simulink library "Lib_EMTAT"  (R2023b)
settings: Solver=VariableStepAuto  StartTime=0.0  StopTime=10.0  RelTol=1e-3
undefined symbols (not defined in the file): MWS
libraries: simulink x34
(part 3 of 4)

== system Lib_EMTAT/Components/Power Flow/AC-DC Rectifier (Efficiency Map)/Open Circuit// Degradation Failure ==
  Eff : Inport
  DegFail? : Inport  Port=2
  OCFail? : Inport  Port=3
  Deg : Inport  Port=4
  Constant : Constant  Value=eps
  Constant1 : Constant
  Divide : Product  Inputs=**
  "If degradation failure, scale Eff." : Switch  Criteria=u2 > Threshold  SaturateOnIntegerOverflow=off  InputSameDT=off
  "If open circuit failure, set Eff = eps." : Switch  Criteria=u2 > Threshold  SaturateOnIntegerOverflow=off  InputSameDT=off
  Sum : Sum  Inputs=+-|
  "Eff " : Outport
  wires:
  DegFail?/1 -> "If degradation failure, scale Eff."/2
  "If degradation failure, scale Eff."/1 -> "If open circuit failure, set Eff = eps."/3
  Divide/1 -> "If degradation failure, scale Eff."/1
  "If open circuit failure, set Eff = eps."/1 -> "Eff "/1
  OCFail?/1 -> "If open circuit failure, set Eff = eps."/2
  Constant/1 -> "If open circuit failure, set Eff = eps."/1
  Sum/1 -> Divide/1
  Eff/1 -> "If degradation failure, scale Eff."/3, Divide/2
  Deg/1 -> Sum/2
  Constant1/1 -> Sum/1

== system Lib_EMTAT/Components/Power Flow/AC-DC Rectifier (Power Loss Map)/Compensate for Divide By Zero. ==
  note: If Vin is not equal to zero, use its value.
      | If Vin is equal to zero, it will calculate a nan value for Iin. Set Iin to zero.
  PEquivAC : Inport
  V_LN_rms : Inport  Port=2
  Fix Divide By Zero. : Subsystem
  I_L_rms : Outport
  wires:
  Fix Divide By Zero./1(I_L_rms) -> I_L_rms/1
  PEquivAC/1 -> Fix Divide By Zero./2(PEquivAC)
  V_LN_rms/1 -> Fix Divide By Zero./1(V_LN_rms)

== system Lib_EMTAT/Components/Power Flow/AC-DC Rectifier (Power Loss Map)/Direction Determination ==
  P_DC : Inport
  Ploss : Inport  Port=2
  Add1 : Sum  Inputs=-+
  Switch : Switch  Criteria=u2 ~= 0  SaturateOnIntegerOverflow=off  InputSameDT=off
  PEquivAC : Outport
  wires:
  P_DC/1 -> Switch/3, Switch/2, Add1/2
  Ploss/1 -> Add1/1
  Add1/1 -> Switch/1
  Switch/1 -> PEquivAC/1

== system Lib_EMTAT/Components/Power Flow/AC-DC Rectifier (Power Loss Map)/Efficiency ==
  P_AC : Inport
  P_DC : Inport  Port=2
  Abs : Abs  SaturateOnIntegerOverflow=off
  Abs1 : Abs  SaturateOnIntegerOverflow=off
  Fix Divide By Zero. : Subsystem
  Fix Divide By Zero.1 : Subsystem
  GreaterThan : RelationalOperator  OutDataTypeStr=boolean  RndMeth=Simplest  InputSameDT=off
  Switch : Switch  Criteria=u2 > Threshold  SaturateOnIntegerOverflow=off  InputSameDT=off
  Eff : Outport
  wires:
  Switch/1 -> Eff/1
  GreaterThan/1 -> Switch/2
  Abs1/1 -> Fix Divide By Zero.1/2(abs(P_AC)), Fix Divide By Zero./1(abs(P_AC)), GreaterThan/2
  P_DC/1 -> Abs/1
  P_AC/1 -> Abs1/1
  Abs/1 -> Fix Divide By Zero.1/1(abs(P_DC)), Fix Divide By Zero./2(abs(P_DC)), GreaterThan/1
  Fix Divide By Zero./1(Eff) -> Switch/3
  Fix Divide By Zero.1/1(Eff) -> Switch/1

== system Lib_EMTAT/Components/Power Flow/AC-DC Rectifier (Power Loss Map)/Failure Determination ==
  Fail? : Inport
  Compare To Constant : simulink/Logic and Bit Operations/Compare To Constant  relop===  const=1  OutDataTypeStr=boolean
  Compare To Constant1 : simulink/Logic and Bit Operations/Compare To Constant  relop===  const=2  OutDataTypeStr=boolean
  Data Type Conversion : DataTypeConversion  OutDataTypeStr=double  SaturateOnIntegerOverflow=off  RndMeth=Floor
  Data Type Conversion1 : DataTypeConversion  OutDataTypeStr=double  SaturateOnIntegerOverflow=off  RndMeth=Floor
  Failure Mode : Constant  Value=FM
  Logical Operator : Logic  AllPortsSameDT=off  OutDataTypeStr=boolean
  Logical Operator1 : Logic  AllPortsSameDT=off  OutDataTypeStr=boolean
  OCFail : Outport
  DegFail : Outport  Port=2
  wires:
  Failure Mode/1 -> Compare To Constant1/1, Compare To Constant/1
  Compare To Constant/1 -> Logical Operator/1
  Logical Operator/1 -> Data Type Conversion/1
  Compare To Constant1/1 -> Logical Operator1/1
  Logical Operator1/1 -> Data Type Conversion1/1
  Fail?/1 -> Logical Operator1/2, Logical Operator/2
  Data Type Conversion1/1 -> DegFail/1
  Data Type Conversion/1 -> OCFail/1

== system Lib_EMTAT/Components/Power Flow/AC-DC Rectifier (Power Loss Map)/Open Circuit Failure - DC Voltage ==
  Failed? : Inport
  V_DC : Inport  Port=2
  Constant : Constant  Value=0
  IsInf : RelationalOperator  Operator=isInf  OutDataTypeStr=boolean  RndMeth=Simplest  InputSameDT=off
  IsNaN : RelationalOperator  Operator=isNaN  OutDataTypeStr=boolean  RndMeth=Simplest  InputSameDT=off
  Logical Operator : Logic  Operator=OR  Inputs=3  AllPortsSameDT=off  OutDataTypeStr=boolean
  Switch : Switch  Criteria=u2 > Threshold  SaturateOnIntegerOverflow=off  InputSameDT=off
  "V_DC " : Outport
  wires:
  Failed?/1 -> Logical Operator/1
  Constant/1 -> Switch/1
  V_DC/1 -> IsNaN/1, IsInf/1, Switch/3
  Switch/1 -> "V_DC "/1
  Logical Operator/1 -> Switch/2
  IsNaN/1 -> Logical Operator/2
  IsInf/1 -> Logical Operator/3

== system Lib_EMTAT/Components/Power Flow/AC-DC Rectifier (Power Loss Map)/Open Circuit// Degradation Failure ==
  Ploss : Inport
  DegFail? : Inport  Port=2
  OCFail? : Inport  Port=3
  Deg : Inport  Port=4
  Constant : Constant  Value=0
  Constant1 : Constant  Value=Plosslim
  Divide : Product  Inputs=**
  "If degradation failure, add to Ploss." : Switch  Criteria=u2 > Threshold  SaturateOnIntegerOverflow=off  InputSameDT=off
  "If open circuit failure, set Ploss = 0." : Switch  Criteria=u2 > Threshold  SaturateOnIntegerOverflow=off  InputSameDT=off
  Sum1 : Sum  Inputs=++|
  "Ploss " : Outport
  wires:
  Divide/1 -> Sum1/1
  Constant1/1 -> Divide/1
  Constant/1 -> "If open circuit failure, set Ploss = 0."/1
  OCFail?/1 -> "If open circuit failure, set Ploss = 0."/2
  "If open circuit failure, set Ploss = 0."/1 -> "Ploss "/1
  Deg/1 -> Divide/2
  Sum1/1 -> "If degradation failure, add to Ploss."/1
  Ploss/1 -> "If degradation failure, add to Ploss."/3, Sum1/2
  "If degradation failure, add to Ploss."/1 -> "If open circuit failure, set Ploss = 0."/3
  DegFail?/1 -> "If degradation failure, add to Ploss."/2

== system Lib_EMTAT/Components/Power Flow/AC-DC Rectifier (Power Loss Map)/Power Loss ==
  V_DC : Inport
  I_L_rms : Inport  Port=2
  2-D Lookup Table : Lookup_n-D  BreakpointsForDimension1=X_C_VoltageInVec_M  BreakpointsForDimension2=Y_C_RMSCurrentOutVec_M  Table=T_C_PowLossArray_M  ExtrapMethod=Clip  UseLastTableValue=on  InternalRulePriority=Speed  RndMeth=Simplest
      settings: InputPortMap=u0,u1
  Abs : Abs  SaturateOnIntegerOverflow=off
  Abs1 : Abs  SaturateOnIntegerOverflow=off
  Saturation : Saturate  UpperLimit=inf  LowerLimit=0
  Ploss : Outport
  wires:
  V_DC/1 -> Abs/1
  Abs/1 -> 2-D Lookup Table/1
  Abs1/1 -> 2-D Lookup Table/2
  I_L_rms/1 -> Abs1/1
  2-D Lookup Table/1 -> Saturation/1
  Saturation/1 -> Ploss/1

== system Lib_EMTAT/Components/Power Flow/Cable/Failure Determination ==
  Fail? : Inport
  OCFail : Outport
  wires:
  Fail?/1 -> OCFail/1

== system Lib_EMTAT/Components/Power Flow/Cable/Fix Zero Voltage Problem ==
  note: If Vin is not equal to zero, pass Vout.
      | If Vin is equal to zero, set Vout to zero. This has to be done because a Vin of 0 would take an efficiency hit and produce a negative Vout.
      | In reality, a zero voltage does not take an efficiency hit.
  "Vout " : Inport
  Vin : Inport  Port=2
  Constant : Constant  Value=0
  Switch : Switch  Criteria=u2 ~= 0  SaturateOnIntegerOverflow=off  InputSameDT=off
  Vout : Outport
  wires:
  Vin/1 -> Switch/2
  "Vout "/1 -> Switch/1
  Constant/1 -> Switch/3
  Switch/1 -> Vout/1

== system Lib_EMTAT/Components/Power Flow/Cable/Open Circuit Failure - Current ==
  Failed? : Inport
  Iin/Iout : Inport  Port=2
  Constant : Constant  Value=0
  IsInf : RelationalOperator  Operator=isInf  OutDataTypeStr=boolean  RndMeth=Simplest  InputSameDT=off
  IsNaN : RelationalOperator  Operator=isNaN  OutDataTypeStr=boolean  RndMeth=Simplest  InputSameDT=off
  Logical Operator : Logic  Operator=OR  Inputs=3  AllPortsSameDT=off  OutDataTypeStr=boolean
  Switch : Switch  Criteria=u2 > Threshold  SaturateOnIntegerOverflow=off  InputSameDT=off
  "Iin/Iout " : Outport
  wires:
  Failed?/1 -> Logical Operator/1
  Constant/1 -> Switch/1
  Iin/Iout/1 -> IsNaN/1, IsInf/1, Switch/3
  Switch/1 -> "Iin/Iout "/1
  Logical Operator/1 -> Switch/2
  IsNaN/1 -> Logical Operator/2
  IsInf/1 -> Logical Operator/3

== system Lib_EMTAT/Components/Power Flow/Cable/Open Circuit Failure - Voltage ==
  Failed? : Inport
  Vout : Inport  Port=2
  Constant : Constant  Value=0
  IsInf : RelationalOperator  Operator=isInf  OutDataTypeStr=boolean  RndMeth=Simplest  InputSameDT=off
  IsNaN : RelationalOperator  Operator=isNaN  OutDataTypeStr=boolean  RndMeth=Simplest  InputSameDT=off
  Logical Operator : Logic  Operator=OR  Inputs=3  AllPortsSameDT=off  OutDataTypeStr=boolean
  Switch : Switch  Criteria=u2 > Threshold  SaturateOnIntegerOverflow=off  InputSameDT=off
  "Vout " : Outport
  wires:
  IsInf/1 -> Logical Operator/3
  IsNaN/1 -> Logical Operator/2
  Logical Operator/1 -> Switch/2
  Switch/1 -> "Vout "/1
  Vout/1 -> Switch/3, IsInf/1, IsNaN/1
  Constant/1 -> Switch/1
  Failed?/1 -> Logical Operator/1

== system Lib_EMTAT/Components/Power Flow/DC-AC Inverter (Efficiency Map)/Compensate for Divide By Zero ==
  note: If Vin is not equal to zero, use its value.
      | If Vin is equal to zero, it will calculate a nan value for Iin. Set Iin to zero.
  PEquivDC : Inport
  V_DC : Inport  Port=2
  Fix Divide By Zero. : Subsystem
  I_DC : Outport
  wires:
  V_DC/1 -> Fix Divide By Zero./1(V_DC)
  PEquivDC/1 -> Fix Divide By Zero./2(PEquivDC)
  Fix Divide By Zero./1(I_DC) -> I_DC/1

== system Lib_EMTAT/Components/Power Flow/DC-AC Inverter (Efficiency Map)/Direction Determination ==
  P_AC : Inport
  Eff : Inport  Port=2
  Divide : Product  Inputs=/*
  Divide1 : Product  Inputs=**
  Switch : Switch  Criteria=u2 > Threshold  SaturateOnIntegerOverflow=off  InputSameDT=off
  PEquivDC : Outport
  wires:
  P_AC/1 -> Divide1/1, Divide/2, Switch/2
  Divide/1 -> Switch/1
  Divide1/1 -> Switch/3
  Eff/1 -> Divide/1, Divide1/2
  Switch/1 -> PEquivDC/1

== system Lib_EMTAT/Components/Power Flow/DC-AC Inverter (Efficiency Map)/Efficiency Table ==
  V_DC : Inport
  I_L_rms : Inport  Port=2
  Abs : Abs  SaturateOnIntegerOverflow=off
  Abs1 : Abs  SaturateOnIntegerOverflow=off
  Efficiency Map : Lookup_n-D  BreakpointsForDimension1=X_C_VoltageInVec_M  BreakpointsForDimension2=Y_C_RMSCurrentOutVec_M  Table=T_C_EffArray_M  ExtrapMethod=Clip  UseLastTableValue=on  InternalRulePriority=Speed  RndMeth=Simplest
      settings: InputPortMap=u0,u1
  Eff : Outport
  wires:
  V_DC/1 -> Abs/1
  Abs/1 -> Efficiency Map/1
  Abs1/1 -> Efficiency Map/2
  I_L_rms/1 -> Abs1/1
  Efficiency Map/1 -> Eff/1

== system Lib_EMTAT/Components/Power Flow/DC-AC Inverter (Efficiency Map)/Failure Determination ==
  Fail? : Inport
  Compare To Constant : simulink/Logic and Bit Operations/Compare To Constant  relop===  const=1  OutDataTypeStr=boolean
  Compare To Constant1 : simulink/Logic and Bit Operations/Compare To Constant  relop===  const=2  OutDataTypeStr=boolean
  Data Type Conversion : DataTypeConversion  OutDataTypeStr=double  SaturateOnIntegerOverflow=off  RndMeth=Floor
  Data Type Conversion1 : DataTypeConversion  OutDataTypeStr=double  SaturateOnIntegerOverflow=off  RndMeth=Floor
  Failure Mode : Constant  Value=FM
  Logical Operator : Logic  AllPortsSameDT=off  OutDataTypeStr=boolean
  Logical Operator1 : Logic  AllPortsSameDT=off  OutDataTypeStr=boolean
  OCFail : Outport
  DegFail : Outport  Port=2
  wires:
  Data Type Conversion/1 -> OCFail/1
  Data Type Conversion1/1 -> DegFail/1
  Fail?/1 -> Logical Operator/2, Logical Operator1/2
  Logical Operator1/1 -> Data Type Conversion1/1
  Compare To Constant1/1 -> Logical Operator1/1
  Logical Operator/1 -> Data Type Conversion/1
  Compare To Constant/1 -> Logical Operator/1
  Failure Mode/1 -> Compare To Constant/1, Compare To Constant1/1

== system Lib_EMTAT/Components/Power Flow/DC-AC Inverter (Efficiency Map)/Open Circuit Failure - DC Current ==
  Failed? : Inport
  I_DC : Inport  Port=2
  Constant : Constant  Value=0
  IsInf : RelationalOperator  Operator=isInf  OutDataTypeStr=boolean  RndMeth=Simplest  InputSameDT=off
  IsNaN : RelationalOperator  Operator=isNaN  OutDataTypeStr=boolean  RndMeth=Simplest  InputSameDT=off
  Logical Operator : Logic  Operator=OR  Inputs=3  AllPortsSameDT=off  OutDataTypeStr=boolean
  Switch : Switch  Criteria=u2 > Threshold  SaturateOnIntegerOverflow=off  InputSameDT=off
  "I_DC " : Outport
  wires:
  Failed?/1 -> Logical Operator/1
  Constant/1 -> Switch/1
  I_DC/1 -> IsNaN/1, IsInf/1, Switch/3
  Switch/1 -> "I_DC "/1
  Logical Operator/1 -> Switch/2
  IsNaN/1 -> Logical Operator/2
  IsInf/1 -> Logical Operator/3

== system Lib_EMTAT/Components/Power Flow/DC-AC Inverter (Efficiency Map)/Open Circuit Failure - Line to Neutral Voltage ==
  Failed? : Inport
  V_LN_rms : Inport  Port=2
  Constant : Constant  Value=0
  IsInf : RelationalOperator  Operator=isInf  OutDataTypeStr=boolean  RndMeth=Simplest  InputSameDT=off
  IsNaN : RelationalOperator  Operator=isNaN  OutDataTypeStr=boolean  RndMeth=Simplest  InputSameDT=off
  Logical Operator : Logic  Operator=OR  Inputs=3  AllPortsSameDT=off  OutDataTypeStr=boolean
  Switch : Switch  Criteria=u2 > Threshold  SaturateOnIntegerOverflow=off  InputSameDT=off
  "V_LN_rms " : Outport
  wires:
  IsInf/1 -> Logical Operator/3
  IsNaN/1 -> Logical Operator/2
  Logical Operator/1 -> Switch/2
  Switch/1 -> "V_LN_rms "/1
  V_LN_rms/1 -> Switch/3, IsInf/1, IsNaN/1
  Constant/1 -> Switch/1
  Failed?/1 -> Logical Operator/1

== system Lib_EMTAT/Components/Power Flow/DC-AC Inverter (Efficiency Map)/Open Circuit// Degradation Failure ==
  Eff : Inport
  DegFail? : Inport  Port=2
  OCFail? : Inport  Port=3
  Deg : Inport  Port=4
  Constant : Constant  Value=eps
  Constant1 : Constant
  Divide : Product  Inputs=**
  "If degradation failure, scale Eff." : Switch  Criteria=u2 > Threshold  SaturateOnIntegerOverflow=off  InputSameDT=off
  "If open circuit failure, set Eff = eps." : Switch  Criteria=u2 > Threshold  SaturateOnIntegerOverflow=off  InputSameDT=off
  Sum : Sum  Inputs=+-|
  "Eff " : Outport
  wires:
  DegFail?/1 -> "If degradation failure, scale Eff."/2
  "If degradation failure, scale Eff."/1 -> "If open circuit failure, set Eff = eps."/3
  Divide/1 -> "If degradation failure, scale Eff."/1
  "If open circuit failure, set Eff = eps."/1 -> "Eff "/1
  OCFail?/1 -> "If open circuit failure, set Eff = eps."/2
  Constant/1 -> "If open circuit failure, set Eff = eps."/1
  Sum/1 -> Divide/1
  Eff/1 -> "If degradation failure, scale Eff."/3, Divide/2
  Deg/1 -> Sum/2
  Constant1/1 -> Sum/1

== system Lib_EMTAT/Components/Power Flow/DC-AC Inverter (Power Loss Map)/Compensate for Divide By Zero ==
  note: If Vin is not equal to zero, use its value.
      | If Vin is equal to zero, it will calculate a nan value for Iin. Set Iin to zero.
  PEquivDC : Inport
  V_DC : Inport  Port=2
  Fix Divide By Zero. : Subsystem
  I_DC : Outport
  wires:
  Fix Divide By Zero./1(I_DC) -> I_DC/1
  PEquivDC/1 -> Fix Divide By Zero./2(PEquivDC)
  V_DC/1 -> Fix Divide By Zero./1(V_DC)

== system Lib_EMTAT/Components/Power Flow/DC-AC Inverter (Power Loss Map)/Direction Determination ==
  P_AC : Inport
  Ploss : Inport  Port=2
  Add1 : Sum
  Switch : Switch  Criteria=u2 ~= 0  SaturateOnIntegerOverflow=off  InputSameDT=off
  PEquivDC : Outport
  wires:
  Add1/1 -> Switch/1
  Ploss/1 -> Add1/1
  P_AC/1 -> Switch/3, Switch/2, Add1/2
  Switch/1 -> PEquivDC/1

== system Lib_EMTAT/Components/Power Flow/DC-AC Inverter (Power Loss Map)/Efficiency ==
  P_AC : Inport
  P_DC : Inport  Port=2
  Abs : Abs  SaturateOnIntegerOverflow=off
  Abs1 : Abs  SaturateOnIntegerOverflow=off
  Fix Divide By Zero. : Subsystem
  Fix Divide By Zero.1 : Subsystem
  GreaterThan : RelationalOperator  OutDataTypeStr=boolean  RndMeth=Simplest  InputSameDT=off
  Switch : Switch  Criteria=u2 > Threshold  SaturateOnIntegerOverflow=off  InputSameDT=off
  Eff : Outport
  wires:
  Switch/1 -> Eff/1
  GreaterThan/1 -> Switch/2
  Abs1/1 -> Fix Divide By Zero.1/2(abs(P_AC)), Fix Divide By Zero./1(abs(P_AC)), GreaterThan/2
  P_DC/1 -> Abs/1
  P_AC/1 -> Abs1/1
  Abs/1 -> Fix Divide By Zero.1/1(abs(P_DC)), Fix Divide By Zero./2(abs(P_DC)), GreaterThan/1
  Fix Divide By Zero./1(Eff) -> Switch/3
  Fix Divide By Zero.1/1(Eff) -> Switch/1

== system Lib_EMTAT/Components/Power Flow/DC-AC Inverter (Power Loss Map)/Failure Determination ==
  Fail? : Inport
  Compare To Constant : simulink/Logic and Bit Operations/Compare To Constant  relop===  const=1  OutDataTypeStr=boolean
  Compare To Constant1 : simulink/Logic and Bit Operations/Compare To Constant  relop===  const=2  OutDataTypeStr=boolean
  Data Type Conversion : DataTypeConversion  OutDataTypeStr=double  SaturateOnIntegerOverflow=off  RndMeth=Floor
  Data Type Conversion1 : DataTypeConversion  OutDataTypeStr=double  SaturateOnIntegerOverflow=off  RndMeth=Floor
  Failure Mode : Constant  Value=FM
  Logical Operator : Logic  AllPortsSameDT=off  OutDataTypeStr=boolean
  Logical Operator1 : Logic  AllPortsSameDT=off  OutDataTypeStr=boolean
  OCFail : Outport
  DegFail : Outport  Port=2
  wires:
  Failure Mode/1 -> Compare To Constant1/1, Compare To Constant/1
  Compare To Constant/1 -> Logical Operator/1
  Logical Operator/1 -> Data Type Conversion/1
  Compare To Constant1/1 -> Logical Operator1/1
  Logical Operator1/1 -> Data Type Conversion1/1
  Fail?/1 -> Logical Operator1/2, Logical Operator/2
  Data Type Conversion1/1 -> DegFail/1
  Data Type Conversion/1 -> OCFail/1

== system Lib_EMTAT/Components/Power Flow/DC-AC Inverter (Power Loss Map)/Open Circuit Failure - DC Current ==
  Failed? : Inport
  I_DC : Inport  Port=2
  Constant : Constant  Value=0
  IsInf : RelationalOperator  Operator=isInf  OutDataTypeStr=boolean  RndMeth=Simplest  InputSameDT=off
  IsNaN : RelationalOperator  Operator=isNaN  OutDataTypeStr=boolean  RndMeth=Simplest  InputSameDT=off
  Logical Operator : Logic  Operator=OR  Inputs=3  AllPortsSameDT=off  OutDataTypeStr=boolean
  Switch : Switch  Criteria=u2 > Threshold  SaturateOnIntegerOverflow=off  InputSameDT=off
  "I_DC " : Outport
  wires:
  IsInf/1 -> Logical Operator/3
  IsNaN/1 -> Logical Operator/2
  Logical Operator/1 -> Switch/2
  Switch/1 -> "I_DC "/1
  I_DC/1 -> Switch/3, IsInf/1, IsNaN/1
  Constant/1 -> Switch/1
  Failed?/1 -> Logical Operator/1

== system Lib_EMTAT/Components/Power Flow/DC-AC Inverter (Power Loss Map)/Open Circuit Failure - Line to Neutral Voltage ==
  Failed? : Inport
  V_LN_rms : Inport  Port=2
  Constant : Constant  Value=0
  IsInf : RelationalOperator  Operator=isInf  OutDataTypeStr=boolean  RndMeth=Simplest  InputSameDT=off
  IsNaN : RelationalOperator  Operator=isNaN  OutDataTypeStr=boolean  RndMeth=Simplest  InputSameDT=off
  Logical Operator : Logic  Operator=OR  Inputs=3  AllPortsSameDT=off  OutDataTypeStr=boolean
  Switch : Switch  Criteria=u2 > Threshold  SaturateOnIntegerOverflow=off  InputSameDT=off
  "V_LN_rms " : Outport
  wires:
  Failed?/1 -> Logical Operator/1
  Constant/1 -> Switch/1
  V_LN_rms/1 -> IsNaN/1, IsInf/1, Switch/3
  Switch/1 -> "V_LN_rms "/1
  Logical Operator/1 -> Switch/2
  IsNaN/1 -> Logical Operator/2
  IsInf/1 -> Logical Operator/3

== system Lib_EMTAT/Components/Power Flow/DC-AC Inverter (Power Loss Map)/Open Circuit// Degradation Failure ==
  Ploss : Inport
  DegFail? : Inport  Port=2
  OCFail? : Inport  Port=3
  Deg : Inport  Port=4
  Constant : Constant  Value=0
  Constant1 : Constant  Value=Plosslim
  Divide : Product  Inputs=**
  "If degradation failure, add to Ploss." : Switch  Criteria=u2 > Threshold  SaturateOnIntegerOverflow=off  InputSameDT=off
  "If open circuit failure, set Ploss = 0." : Switch  Criteria=u2 > Threshold  SaturateOnIntegerOverflow=off  InputSameDT=off
  Sum1 : Sum  Inputs=++|
  "Ploss " : Outport
  wires:
  Divide/1 -> Sum1/1
  Constant1/1 -> Divide/1
  Constant/1 -> "If open circuit failure, set Ploss = 0."/1
  OCFail?/1 -> "If open circuit failure, set Ploss = 0."/2
  "If open circuit failure, set Ploss = 0."/1 -> "Ploss "/1
  Deg/1 -> Divide/2
  Sum1/1 -> "If degradation failure, add to Ploss."/1
  Ploss/1 -> "If degradation failure, add to Ploss."/3, Sum1/2
  "If degradation failure, add to Ploss."/1 -> "If open circuit failure, set Ploss = 0."/3
  DegFail?/1 -> "If degradation failure, add to Ploss."/2

== system Lib_EMTAT/Components/Power Flow/DC-AC Inverter (Power Loss Map)/Power Loss ==
  V_DC : Inport
  I_L_rms : Inport  Port=2
  2-D Lookup Table : Lookup_n-D  BreakpointsForDimension1=X_C_VoltageInVec_M  BreakpointsForDimension2=Y_C_RMSCurrentOutVec_M  Table=T_C_PowLossArray_M  ExtrapMethod=Clip  UseLastTableValue=on  InternalRulePriority=Speed  RndMeth=Simplest
      settings: InputPortMap=u0,u1
  Abs : Abs  SaturateOnIntegerOverflow=off
  Abs1 : Abs  SaturateOnIntegerOverflow=off
  Saturation : Saturate  UpperLimit=inf  LowerLimit=0
  Ploss : Outport
  wires:
  Saturation/1 -> Ploss/1
  2-D Lookup Table/1 -> Saturation/1
  I_L_rms/1 -> Abs1/1
  Abs1/1 -> 2-D Lookup Table/2
  Abs/1 -> 2-D Lookup Table/1
  V_DC/1 -> Abs/1

== system Lib_EMTAT/Components/Power Flow/DC-DC Converter (Efficiency Map) (Regulate Output Voltage)/Compensate for Divide By Zero ==
  note: If Vin is not equal to zero, use its value.
      | If Vin is equal to zero, it will calculate a nan value for Iin. Set Iin to zero.
  Pin : Inport
  Vin : Inport  Port=2
  Fix Divide By Zero. : Subsystem
  Iin : Outport
  wires:
  Fix Divide By Zero./1(Iin) -> Iin/1
  Pin/1 -> Fix Divide By Zero./2(Pin)
  Vin/1 -> Fix Divide By Zero./1(Vin)

== system Lib_EMTAT/Components/Power Flow/DC-DC Converter (Efficiency Map) (Regulate Output Voltage)/Direction Determination ==
  Pout : Inport
  Eff : Inport  Port=2
  Divide : Product  Inputs=/*
  Divide1 : Product  Inputs=**
  Switch : Switch  Criteria=u2 > Threshold  SaturateOnIntegerOverflow=off  InputSameDT=off
  Pin : Outport
  wires:
  Pout/1 -> Divide1/1, Divide/2, Switch/2
  Divide/1 -> Switch/1
  Divide1/1 -> Switch/3
  Eff/1 -> Divide/1, Divide1/2
  Switch/1 -> Pin/1

== system Lib_EMTAT/Components/Power Flow/DC-DC Converter (Efficiency Map) (Regulate Output Voltage)/Efficiency ==
  Vin : Inport
  Iout : Inport  Port=2
  2-D Lookup Table : Lookup_n-D  BreakpointsForDimension1=X_Vin_VoltageVec_M  BreakpointsForDimension2=Y_Iout_CurrentVec_M  Table=T_C_EffArray_M  ExtrapMethod=Clip  UseLastTableValue=on  InternalRulePriority=Speed  RndMeth=Simplest
      settings: InputPortMap=u0,u1
  Abs : Abs  SaturateOnIntegerOverflow=off
  Abs1 : Abs  SaturateOnIntegerOverflow=off
  Eff : Outport
  wires:
  Vin/1 -> Abs/1
  Abs/1 -> 2-D Lookup Table/1
  Abs1/1 -> 2-D Lookup Table/2
  Iout/1 -> Abs1/1
  2-D Lookup Table/1 -> Eff/1

== system Lib_EMTAT/Components/Power Flow/DC-DC Converter (Efficiency Map) (Regulate Output Voltage)/Failure Determination ==
  Fail? : Inport
  Compare To Constant : simulink/Logic and Bit Operations/Compare To Constant  relop===  const=1  OutDataTypeStr=boolean
  Compare To Constant1 : simulink/Logic and Bit Operations/Compare To Constant  relop===  const=2  OutDataTypeStr=boolean
  Data Type Conversion : DataTypeConversion  OutDataTypeStr=double  SaturateOnIntegerOverflow=off  RndMeth=Floor
  Data Type Conversion1 : DataTypeConversion  OutDataTypeStr=double  SaturateOnIntegerOverflow=off  RndMeth=Floor
  Failure Mode : Constant  Value=FM
  Logical Operator : Logic  AllPortsSameDT=off  OutDataTypeStr=boolean
  Logical Operator1 : Logic  AllPortsSameDT=off  OutDataTypeStr=boolean
  OCFail : Outport
  DegFail : Outport  Port=2
  wires:
  Data Type Conversion/1 -> OCFail/1
  Data Type Conversion1/1 -> DegFail/1
  Fail?/1 -> Logical Operator/2, Logical Operator1/2
  Logical Operator1/1 -> Data Type Conversion1/1
  Compare To Constant1/1 -> Logical Operator1/1
  Logical Operator/1 -> Data Type Conversion/1
  Compare To Constant/1 -> Logical Operator/1
  Failure Mode/1 -> Compare To Constant/1, Compare To Constant1/1

== system Lib_EMTAT/Components/Power Flow/DC-DC Converter (Efficiency Map) (Regulate Output Voltage)/Open Circuit Failure - Input Current ==
  Failed? : Inport
  Iin : Inport  Port=2
  Constant : Constant  Value=0
  IsInf : RelationalOperator  Operator=isInf  OutDataTypeStr=boolean  RndMeth=Simplest  InputSameDT=off
  IsNaN : RelationalOperator  Operator=isNaN  OutDataTypeStr=boolean  RndMeth=Simplest  InputSameDT=off
  Logical Operator : Logic  Operator=OR  Inputs=3  AllPortsSameDT=off  OutDataTypeStr=boolean
  Switch : Switch  Criteria=u2 > Threshold  SaturateOnIntegerOverflow=off  InputSameDT=off
  "Iin  " : Outport
  wires:
  IsInf/1 -> Logical Operator/3
  IsNaN/1 -> Logical Operator/2
  Logical Operator/1 -> Switch/2
  Switch/1 -> "Iin  "/1
  Iin/1 -> Switch/3, IsInf/1, IsNaN/1
  Constant/1 -> Switch/1
  Failed?/1 -> Logical Operator/1

== system Lib_EMTAT/Components/Power Flow/DC-DC Converter (Efficiency Map) (Regulate Output Voltage)/Open Circuit Failure - Output Voltage ==
  Failed? : Inport
  Vout : Inport  Port=2
  Constant : Constant  Value=0
  IsInf : RelationalOperator  Operator=isInf  OutDataTypeStr=boolean  RndMeth=Simplest  InputSameDT=off
  IsNaN : RelationalOperator  Operator=isNaN  OutDataTypeStr=boolean  RndMeth=Simplest  InputSameDT=off
  Logical Operator : Logic  Operator=OR  Inputs=3  AllPortsSameDT=off  OutDataTypeStr=boolean
  Switch : Switch  Criteria=u2 > Threshold  SaturateOnIntegerOverflow=off  InputSameDT=off
  "Vout   " : Outport
  wires:
  Failed?/1 -> Logical Operator/1
  Constant/1 -> Switch/1
  Vout/1 -> IsNaN/1, IsInf/1, Switch/3
  Switch/1 -> "Vout   "/1
  Logical Operator/1 -> Switch/2
  IsNaN/1 -> Logical Operator/2
  IsInf/1 -> Logical Operator/3

== system Lib_EMTAT/Components/Power Flow/DC-DC Converter (Efficiency Map) (Regulate Output Voltage)/Open Circuit// Degradation Failure ==
  Eff : Inport
  DegFail? : Inport  Port=2
  OCFail? : Inport  Port=3
  Deg : Inport  Port=4
  Constant : Constant  Value=eps
  Constant1 : Constant
  Divide : Product  Inputs=**
  "If degradation failure, scale Eff." : Switch  Criteria=u2 > Threshold  SaturateOnIntegerOverflow=off  InputSameDT=off
  "If open circuit failure, set Eff = eps." : Switch  Criteria=u2 > Threshold  SaturateOnIntegerOverflow=off  InputSameDT=off
  Sum : Sum  Inputs=+-|
  "Eff " : Outport
  wires:
  DegFail?/1 -> "If degradation failure, scale Eff."/2
  "If degradation failure, scale Eff."/1 -> "If open circuit failure, set Eff = eps."/3
  Divide/1 -> "If degradation failure, scale Eff."/1
  "If open circuit failure, set Eff = eps."/1 -> "Eff "/1
  OCFail?/1 -> "If open circuit failure, set Eff = eps."/2
  Constant/1 -> "If open circuit failure, set Eff = eps."/1
  Sum/1 -> Divide/1
  Eff/1 -> "If degradation failure, scale Eff."/3, Divide/2
  Deg/1 -> Sum/2
  Constant1/1 -> Sum/1

== system Lib_EMTAT/Components/Power Flow/DC-DC Converter (Efficiency Map) (Set Output Voltage)/Compensate for Divide By Zero ==
  note: If Vin is not equal to zero, use its value.
      | If Vin is equal to zero, it will calculate a nan value for Iin. Set Iin to zero.
  Pin : Inport
  Vin : Inport  Port=2
  Fix Divide By Zero. : Subsystem
  Iin : Outport
  wires:
  Vin/1 -> Fix Divide By Zero./1(Vin)
  Pin/1 -> Fix Divide By Zero./2(Pin)
  Fix Divide By Zero./1(Iin) -> Iin/1

== system Lib_EMTAT/Components/Power Flow/DC-DC Converter (Efficiency Map) (Set Output Voltage)/Direction Determination ==
  Pout : Inport
  Eff : Inport  Port=2
  Divide : Product  Inputs=/*
  Divide1 : Product  Inputs=**
  Switch : Switch  Criteria=u2 > Threshold  SaturateOnIntegerOverflow=off  InputSameDT=off
  Pin : Outport
  wires:
  Pout/1 -> Divide1/1, Divide/2, Switch/2
  Divide/1 -> Switch/1
  Divide1/1 -> Switch/3
  Eff/1 -> Divide/1, Divide1/2
  Switch/1 -> Pin/1

== system Lib_EMTAT/Components/Power Flow/DC-DC Converter (Efficiency Map) (Set Output Voltage)/Efficiency ==
  Vin : Inport
  Iout : Inport  Port=2
  2-D Lookup Table : Lookup_n-D  BreakpointsForDimension1=X_Vin_VoltageVec_M  BreakpointsForDimension2=Y_Iout_CurrentVec_M  Table=T_C_EffArray_M  ExtrapMethod=Clip  UseLastTableValue=on  InternalRulePriority=Speed  RndMeth=Simplest
      settings: InputPortMap=u0,u1
  Abs : Abs  SaturateOnIntegerOverflow=off
  Abs1 : Abs  SaturateOnIntegerOverflow=off
  Eff : Outport
  wires:
  2-D Lookup Table/1 -> Eff/1
  Iout/1 -> Abs1/1
  Abs1/1 -> 2-D Lookup Table/2
  Abs/1 -> 2-D Lookup Table/1
  Vin/1 -> Abs/1

== system Lib_EMTAT/Components/Power Flow/DC-DC Converter (Efficiency Map) (Set Output Voltage)/Failure Determination ==
  Fail? : Inport
  Compare To Constant : simulink/Logic and Bit Operations/Compare To Constant  relop===  const=1  OutDataTypeStr=boolean
  Compare To Constant1 : simulink/Logic and Bit Operations/Compare To Constant  relop===  const=2  OutDataTypeStr=boolean
  Data Type Conversion : DataTypeConversion  OutDataTypeStr=double  SaturateOnIntegerOverflow=off  RndMeth=Floor
  Data Type Conversion1 : DataTypeConversion  OutDataTypeStr=double  SaturateOnIntegerOverflow=off  RndMeth=Floor
  Failure Mode : Constant  Value=FM
  Logical Operator : Logic  AllPortsSameDT=off  OutDataTypeStr=boolean
  Logical Operator1 : Logic  AllPortsSameDT=off  OutDataTypeStr=boolean
  OCFail : Outport
  DegFail : Outport  Port=2
  wires:
  Failure Mode/1 -> Compare To Constant1/1, Compare To Constant/1
  Compare To Constant/1 -> Logical Operator/1
  Logical Operator/1 -> Data Type Conversion/1
  Compare To Constant1/1 -> Logical Operator1/1
  Logical Operator1/1 -> Data Type Conversion1/1
  Fail?/1 -> Logical Operator1/2, Logical Operator/2
  Data Type Conversion1/1 -> DegFail/1
  Data Type Conversion/1 -> OCFail/1

== system Lib_EMTAT/Components/Power Flow/DC-DC Converter (Efficiency Map) (Set Output Voltage)/Open Circuit Failure - Input Current ==
  Failed? : Inport
  Iin : Inport  Port=2
  Constant : Constant  Value=0
  IsInf : RelationalOperator  Operator=isInf  OutDataTypeStr=boolean  RndMeth=Simplest  InputSameDT=off
  IsNaN : RelationalOperator  Operator=isNaN  OutDataTypeStr=boolean  RndMeth=Simplest  InputSameDT=off
  Logical Operator : Logic  Operator=OR  Inputs=3  AllPortsSameDT=off  OutDataTypeStr=boolean
  Switch : Switch  Criteria=u2 > Threshold  SaturateOnIntegerOverflow=off  InputSameDT=off
  "Iin  " : Outport
  wires:
  Failed?/1 -> Logical Operator/1
  Constant/1 -> Switch/1
  Iin/1 -> IsNaN/1, IsInf/1, Switch/3
  Switch/1 -> "Iin  "/1
  Logical Operator/1 -> Switch/2
  IsNaN/1 -> Logical Operator/2
  IsInf/1 -> Logical Operator/3

== system Lib_EMTAT/Components/Power Flow/DC-DC Converter (Efficiency Map) (Set Output Voltage)/Open Circuit Failure - Output Voltage ==
  Failed? : Inport
  Vout : Inport  Port=2
  Constant : Constant  Value=0
  IsInf : RelationalOperator  Operator=isInf  OutDataTypeStr=boolean  RndMeth=Simplest  InputSameDT=off
  IsNaN : RelationalOperator  Operator=isNaN  OutDataTypeStr=boolean  RndMeth=Simplest  InputSameDT=off
  Logical Operator : Logic  Operator=OR  Inputs=3  AllPortsSameDT=off  OutDataTypeStr=boolean
  Switch : Switch  Criteria=u2 > Threshold  SaturateOnIntegerOverflow=off  InputSameDT=off
  "Vout   " : Outport
  wires:
  IsInf/1 -> Logical Operator/3
  IsNaN/1 -> Logical Operator/2
  Logical Operator/1 -> Switch/2
  Switch/1 -> "Vout   "/1
  Vout/1 -> Switch/3, IsInf/1, IsNaN/1
  Constant/1 -> Switch/1
  Failed?/1 -> Logical Operator/1

== system Lib_EMTAT/Components/Power Flow/DC-DC Converter (Efficiency Map) (Set Output Voltage)/Open Circuit// Degradation Failure ==
  Eff : Inport
  DegFail? : Inport  Port=2
  OCFail? : Inport  Port=3
  Deg : Inport  Port=4
  Constant : Constant  Value=eps
  Constant1 : Constant
  Divide : Product  Inputs=**
  "If degradation failure, scale Eff." : Switch  Criteria=u2 > Threshold  SaturateOnIntegerOverflow=off  InputSameDT=off
  "If open circuit failure, set Eff = eps." : Switch  Criteria=u2 > Threshold  SaturateOnIntegerOverflow=off  InputSameDT=off
  Sum : Sum  Inputs=+-|
  "Eff " : Outport
  wires:
  DegFail?/1 -> "If degradation failure, scale Eff."/2
  "If degradation failure, scale Eff."/1 -> "If open circuit failure, set Eff = eps."/3
  Divide/1 -> "If degradation failure, scale Eff."/1
  "If open circuit failure, set Eff = eps."/1 -> "Eff "/1
  OCFail?/1 -> "If open circuit failure, set Eff = eps."/2
  Constant/1 -> "If open circuit failure, set Eff = eps."/1
  Sum/1 -> Divide/1
  Eff/1 -> "If degradation failure, scale Eff."/3, Divide/2
  Deg/1 -> Sum/2
  Constant1/1 -> Sum/1

== system Lib_EMTAT/Components/Power Flow/DC-DC Converter (Power Loss Map) (Regulate Output Voltage)/Compensate for Divide By Zero ==
  note: If Vin is not equal to zero, use its value.
      | If Vin is equal to zero, it will calculate a nan value for Iin. Set Iin to zero.
  Pin : Inport
  Vin : Inport  Port=2
  Fix Divide By Zero. : Subsystem
  Iin : Outport
  wires:
  Vin/1 -> Fix Divide By Zero./1(Vin)
  Pin/1 -> Fix Divide By Zero./2(Pin)
  Fix Divide By Zero./1(Iin) -> Iin/1

== system Lib_EMTAT/Components/Power Flow/DC-DC Converter (Power Loss Map) (Regulate Output Voltage)/Direction Determination ==
  Pout : Inport
  Ploss : Inport  Port=2
  Add1 : Sum
  Switch : Switch  Criteria=u2 ~= 0  SaturateOnIntegerOverflow=off  InputSameDT=off
  Pin : Outport
  wires:
  Add1/1 -> Switch/1
  Ploss/1 -> Add1/1
  Pout/1 -> Switch/3, Switch/2, Add1/2
  Switch/1 -> Pin/1

== system Lib_EMTAT/Components/Power Flow/DC-DC Converter (Power Loss Map) (Regulate Output Voltage)/Efficiency ==
  Pout : Inport
  Pin : Inport  Port=2
  Abs : Abs  SaturateOnIntegerOverflow=off
  Abs1 : Abs  SaturateOnIntegerOverflow=off
  Fix Divide By Zero. : Subsystem
  Fix Divide By Zero.1 : Subsystem
  GreaterThan : RelationalOperator  OutDataTypeStr=boolean  RndMeth=Simplest  InputSameDT=off
  Switch : Switch  Criteria=u2 > Threshold  SaturateOnIntegerOverflow=off  InputSameDT=off
  Eff : Outport
  wires:
  Switch/1 -> Eff/1
  GreaterThan/1 -> Switch/2
  Abs1/1 -> Fix Divide By Zero.1/2(abs(Pout)), Fix Divide By Zero./1(abs(Pout)), GreaterThan/2
  Pin/1 -> Abs/1
  Pout/1 -> Abs1/1
  Abs/1 -> Fix Divide By Zero.1/1(abs(Pin)), Fix Divide By Zero./2(abs(Pin)), GreaterThan/1
  Fix Divide By Zero./1(Eff) -> Switch/3
  Fix Divide By Zero.1/1(Eff) -> Switch/1

== system Lib_EMTAT/Components/Power Flow/DC-DC Converter (Power Loss Map) (Regulate Output Voltage)/Failure Determination ==
  Fail? : Inport
  Compare To Constant : simulink/Logic and Bit Operations/Compare To Constant  relop===  const=1  OutDataTypeStr=boolean
  Compare To Constant1 : simulink/Logic and Bit Operations/Compare To Constant  relop===  const=2  OutDataTypeStr=boolean
  Data Type Conversion : DataTypeConversion  OutDataTypeStr=double  SaturateOnIntegerOverflow=off  RndMeth=Floor
  Data Type Conversion1 : DataTypeConversion  OutDataTypeStr=double  SaturateOnIntegerOverflow=off  RndMeth=Floor
  Failure Mode : Constant  Value=FM
  Logical Operator : Logic  AllPortsSameDT=off  OutDataTypeStr=boolean
  Logical Operator1 : Logic  AllPortsSameDT=off  OutDataTypeStr=boolean
  OCFail : Outport
  DegFail : Outport  Port=2
  wires:
  Failure Mode/1 -> Compare To Constant1/1, Compare To Constant/1
  Compare To Constant/1 -> Logical Operator/1
  Logical Operator/1 -> Data Type Conversion/1
  Compare To Constant1/1 -> Logical Operator1/1
  Logical Operator1/1 -> Data Type Conversion1/1
  Fail?/1 -> Logical Operator1/2, Logical Operator/2
  Data Type Conversion1/1 -> DegFail/1
  Data Type Conversion/1 -> OCFail/1

== system Lib_EMTAT/Components/Power Flow/DC-DC Converter (Power Loss Map) (Regulate Output Voltage)/Open Circuit Failure - Input Current ==
  Failed? : Inport
  Iin : Inport  Port=2
  Constant : Constant  Value=0
  IsInf : RelationalOperator  Operator=isInf  OutDataTypeStr=boolean  RndMeth=Simplest  InputSameDT=off
  IsNaN : RelationalOperator  Operator=isNaN  OutDataTypeStr=boolean  RndMeth=Simplest  InputSameDT=off
  Logical Operator : Logic  Operator=OR  Inputs=3  AllPortsSameDT=off  OutDataTypeStr=boolean
  Switch : Switch  Criteria=u2 > Threshold  SaturateOnIntegerOverflow=off  InputSameDT=off
  "Iin  " : Outport
  wires:
  Failed?/1 -> Logical Operator/1
  Constant/1 -> Switch/1
  Iin/1 -> IsNaN/1, IsInf/1, Switch/3
  Switch/1 -> "Iin  "/1
  Logical Operator/1 -> Switch/2
  IsNaN/1 -> Logical Operator/2
  IsInf/1 -> Logical Operator/3

== system Lib_EMTAT/Components/Power Flow/DC-DC Converter (Power Loss Map) (Regulate Output Voltage)/Open Circuit Failure - Output Voltage ==
  Failed? : Inport
  Vout : Inport  Port=2
  Constant : Constant  Value=0
  IsInf : RelationalOperator  Operator=isInf  OutDataTypeStr=boolean  RndMeth=Simplest  InputSameDT=off
  IsNaN : RelationalOperator  Operator=isNaN  OutDataTypeStr=boolean  RndMeth=Simplest  InputSameDT=off
  Logical Operator : Logic  Operator=OR  Inputs=3  AllPortsSameDT=off  OutDataTypeStr=boolean
  Switch : Switch  Criteria=u2 > Threshold  SaturateOnIntegerOverflow=off  InputSameDT=off
  "Vout   " : Outport
  wires:
  IsInf/1 -> Logical Operator/3
  IsNaN/1 -> Logical Operator/2
  Logical Operator/1 -> Switch/2
  Switch/1 -> "Vout   "/1
  Vout/1 -> Switch/3, IsInf/1, IsNaN/1
  Constant/1 -> Switch/1
  Failed?/1 -> Logical Operator/1

== system Lib_EMTAT/Components/Power Flow/DC-DC Converter (Power Loss Map) (Regulate Output Voltage)/Open Circuit// Degradation Failure ==
  Ploss : Inport
  DegFail? : Inport  Port=2
  OCFail? : Inport  Port=3
  Deg : Inport  Port=4
  Constant : Constant  Value=0
  Constant1 : Constant  Value=Plosslim
  Divide : Product  Inputs=**
  "If degradation failure, add to Ploss." : Switch  Criteria=u2 > Threshold  SaturateOnIntegerOverflow=off  InputSameDT=off
  "If open circuit failure, set Ploss = 0." : Switch  Criteria=u2 > Threshold  SaturateOnIntegerOverflow=off  InputSameDT=off
  Sum1 : Sum  Inputs=++|
  "Ploss " : Outport
  wires:
  DegFail?/1 -> "If degradation failure, add to Ploss."/2
  "If degradation failure, add to Ploss."/1 -> "If open circuit failure, set Ploss = 0."/3
  Ploss/1 -> Sum1/2, "If degradation failure, add to Ploss."/3
  Sum1/1 -> "If degradation failure, add to Ploss."/1
  Deg/1 -> Divide/2
  "If open circuit failure, set Ploss = 0."/1 -> "Ploss "/1
  OCFail?/1 -> "If open circuit failure, set Ploss = 0."/2
  Constant/1 -> "If open circuit failure, set Ploss = 0."/1
  Constant1/1 -> Divide/1
  Divide/1 -> Sum1/1

== system Lib_EMTAT/Components/Power Flow/DC-DC Converter (Power Loss Map) (Regulate Output Voltage)/Power Loss ==
  Vin : Inport
  Iout : Inport  Port=2
  2-D Lookup Table : Lookup_n-D  BreakpointsForDimension1=X_Vin_VoltageVec_M  BreakpointsForDimension2=Y_Iout_CurrentVec_M  Table=T_C_PlossArray_M  ExtrapMethod=Clip  UseLastTableValue=on  InternalRulePriority=Speed  RndMeth=Simplest
      settings: InputPortMap=u0,u1
  Abs : Abs  SaturateOnIntegerOverflow=off
  Abs1 : Abs  SaturateOnIntegerOverflow=off
  Ploss : Outport
  wires:
  2-D Lookup Table/1 -> Ploss/1
  Iout/1 -> Abs1/1
  Abs1/1 -> 2-D Lookup Table/2
  Abs/1 -> 2-D Lookup Table/1
  Vin/1 -> Abs/1

== system Lib_EMTAT/Components/Power Flow/DC-DC Converter (Power Loss Map) (Set Output Voltage)/Compensate for Divide By Zero ==
  note: If Vin is not equal to zero, use its value.
      | If Vin is equal to zero, it will calculate a nan value for Iin. Set Iin to zero.
  Pin : Inport
  Vin : Inport  Port=2
  Fix Divide By Zero. : Subsystem
  Iin : Outport
  wires:
  Fix Divide By Zero./1(Iin) -> Iin/1
  Pin/1 -> Fix Divide By Zero./2(Pin)
  Vin/1 -> Fix Divide By Zero./1(Vin)

== system Lib_EMTAT/Components/Power Flow/DC-DC Converter (Power Loss Map) (Set Output Voltage)/Direction Determination ==
  Pout : Inport
  Ploss : Inport  Port=2
  Add1 : Sum
  Switch : Switch  Criteria=u2 ~= 0  SaturateOnIntegerOverflow=off  InputSameDT=off
  Pin : Outport
  wires:
  Switch/1 -> Pin/1
  Pout/1 -> Add1/2, Switch/2, Switch/3
  Ploss/1 -> Add1/1
  Add1/1 -> Switch/1

== system Lib_EMTAT/Components/Power Flow/DC-DC Converter (Power Loss Map) (Set Output Voltage)/Efficiency ==
  Pout : Inport
  Pin : Inport  Port=2
  Abs : Abs  SaturateOnIntegerOverflow=off
  Abs1 : Abs  SaturateOnIntegerOverflow=off
  Fix Divide By Zero. : Subsystem
  Fix Divide By Zero.1 : Subsystem
  GreaterThan : RelationalOperator  OutDataTypeStr=boolean  RndMeth=Simplest  InputSameDT=off
  Switch : Switch  Criteria=u2 > Threshold  SaturateOnIntegerOverflow=off  InputSameDT=off
  Eff : Outport
  wires:
  Fix Divide By Zero.1/1(Eff) -> Switch/1
  Fix Divide By Zero./1(Eff) -> Switch/3
  Abs/1 -> GreaterThan/1, Fix Divide By Zero./2(abs(Pin)), Fix Divide By Zero.1/1(abs(Pin))
  Pout/1 -> Abs1/1
  Pin/1 -> Abs/1
  Abs1/1 -> GreaterThan/2, Fix Divide By Zero./1(abs(Pout)), Fix Divide By Zero.1/2(abs(Pout))
  GreaterThan/1 -> Switch/2
  Switch/1 -> Eff/1

== system Lib_EMTAT/Components/Power Flow/DC-DC Converter (Power Loss Map) (Set Output Voltage)/Failure Determination ==
  Fail? : Inport
  Compare To Constant : simulink/Logic and Bit Operations/Compare To Constant  relop===  const=1  OutDataTypeStr=boolean
  Compare To Constant1 : simulink/Logic and Bit Operations/Compare To Constant  relop===  const=2  OutDataTypeStr=boolean
  Data Type Conversion : DataTypeConversion  OutDataTypeStr=double  SaturateOnIntegerOverflow=off  RndMeth=Floor
  Data Type Conversion1 : DataTypeConversion  OutDataTypeStr=double  SaturateOnIntegerOverflow=off  RndMeth=Floor
  Failure Mode : Constant  Value=FM
  Logical Operator : Logic  AllPortsSameDT=off  OutDataTypeStr=boolean
  Logical Operator1 : Logic  AllPortsSameDT=off  OutDataTypeStr=boolean
  OCFail : Outport
  DegFail : Outport  Port=2
  wires:
  Data Type Conversion/1 -> OCFail/1
  Data Type Conversion1/1 -> DegFail/1
  Fail?/1 -> Logical Operator/2, Logical Operator1/2
  Logical Operator1/1 -> Data Type Conversion1/1
  Compare To Constant1/1 -> Logical Operator1/1
  Logical Operator/1 -> Data Type Conversion/1
  Compare To Constant/1 -> Logical Operator/1
  Failure Mode/1 -> Compare To Constant/1, Compare To Constant1/1

== system Lib_EMTAT/Components/Power Flow/DC-DC Converter (Power Loss Map) (Set Output Voltage)/Open Circuit Failure - Input Current ==
  Failed? : Inport
  Iin : Inport  Port=2
  Constant : Constant  Value=0
  IsInf : RelationalOperator  Operator=isInf  OutDataTypeStr=boolean  RndMeth=Simplest  InputSameDT=off
  IsNaN : RelationalOperator  Operator=isNaN  OutDataTypeStr=boolean  RndMeth=Simplest  InputSameDT=off
  Logical Operator : Logic  Operator=OR  Inputs=3  AllPortsSameDT=off  OutDataTypeStr=boolean
  Switch : Switch  Criteria=u2 > Threshold  SaturateOnIntegerOverflow=off  InputSameDT=off
  "Iin  " : Outport
  wires:
  IsInf/1 -> Logical Operator/3
  IsNaN/1 -> Logical Operator/2
  Logical Operator/1 -> Switch/2
  Switch/1 -> "Iin  "/1
  Iin/1 -> Switch/3, IsInf/1, IsNaN/1
  Constant/1 -> Switch/1
  Failed?/1 -> Logical Operator/1

== system Lib_EMTAT/Components/Power Flow/DC-DC Converter (Power Loss Map) (Set Output Voltage)/Open Circuit Failure - Output Voltage ==
  Failed? : Inport
  Vout : Inport  Port=2
  Constant : Constant  Value=0
  IsInf : RelationalOperator  Operator=isInf  OutDataTypeStr=boolean  RndMeth=Simplest  InputSameDT=off
  IsNaN : RelationalOperator  Operator=isNaN  OutDataTypeStr=boolean  RndMeth=Simplest  InputSameDT=off
  Logical Operator : Logic  Operator=OR  Inputs=3  AllPortsSameDT=off  OutDataTypeStr=boolean
  Switch : Switch  Criteria=u2 > Threshold  SaturateOnIntegerOverflow=off  InputSameDT=off
  "Vout   " : Outport
  wires:
  Failed?/1 -> Logical Operator/1
  Constant/1 -> Switch/1
  Vout/1 -> IsNaN/1, IsInf/1, Switch/3
  Switch/1 -> "Vout   "/1
  Logical Operator/1 -> Switch/2
  IsNaN/1 -> Logical Operator/2
  IsInf/1 -> Logical Operator/3

== system Lib_EMTAT/Components/Power Flow/DC-DC Converter (Power Loss Map) (Set Output Voltage)/Open Circuit// Degradation Failure ==
  Ploss : Inport
  DegFail? : Inport  Port=2
  OCFail? : Inport  Port=3
  Deg : Inport  Port=4
  Constant : Constant  Value=0
  Constant1 : Constant  Value=Plosslim
  Divide : Product  Inputs=**
  "If degradation failure, add to Ploss." : Switch  Criteria=u2 > Threshold  SaturateOnIntegerOverflow=off  InputSameDT=off
  "If open circuit failure, set Ploss = 0." : Switch  Criteria=u2 > Threshold  SaturateOnIntegerOverflow=off  InputSameDT=off
  Sum1 : Sum  Inputs=++|
  "Ploss " : Outport
  wires:
  Divide/1 -> Sum1/1
  Constant1/1 -> Divide/1
  Constant/1 -> "If open circuit failure, set Ploss = 0."/1
  OCFail?/1 -> "If open circuit failure, set Ploss = 0."/2
  "If open circuit failure, set Ploss = 0."/1 -> "Ploss "/1
  Deg/1 -> Divide/2
  Sum1/1 -> "If degradation failure, add to Ploss."/1
  Ploss/1 -> "If degradation failure, add to Ploss."/3, Sum1/2
  "If degradation failure, add to Ploss."/1 -> "If open circuit failure, set Ploss = 0."/3
  DegFail?/1 -> "If degradation failure, add to Ploss."/2

== system Lib_EMTAT/Components/Power Flow/DC-DC Converter (Power Loss Map) (Set Output Voltage)/Power Loss ==
  Vin : Inport
  Iout : Inport  Port=2
  2-D Lookup Table : Lookup_n-D  BreakpointsForDimension1=X_Vin_VoltageVec_M  BreakpointsForDimension2=Y_Iout_CurrentVec_M  Table=T_C_PlossArray_M  ExtrapMethod=Clip  UseLastTableValue=on  InternalRulePriority=Speed  RndMeth=Simplest
      settings: InputPortMap=u0,u1
  Abs : Abs  SaturateOnIntegerOverflow=off
  Abs1 : Abs  SaturateOnIntegerOverflow=off
  Ploss : Outport
  wires:
  Vin/1 -> Abs/1
  Abs/1 -> 2-D Lookup Table/1
  Abs1/1 -> 2-D Lookup Table/2
  Iout/1 -> Abs1/1
  2-D Lookup Table/1 -> Ploss/1

== system Lib_EMTAT/Components/Power Flow/Mechanical Shaft/Failure Determination ==
  Fail? : Inport
  SBFail : Outport
  wires:
  Fail?/1 -> SBFail/1

== system Lib_EMTAT/Components/Power Flow/Mechanical Shaft/Shaft Break Failure ==
  Failed? : Inport
  T : Inport  Port=2
  Constant : Constant  Value=0
  IsInf : RelationalOperator  Operator=isInf  OutDataTypeStr=boolean  RndMeth=Simplest  InputSameDT=off
  IsNaN : RelationalOperator  Operator=isNaN  OutDataTypeStr=boolean  RndMeth=Simplest  InputSameDT=off
  Logical Operator : Logic  Operator=OR  Inputs=3  AllPortsSameDT=off  OutDataTypeStr=boolean
  Switch : Switch  Criteria=u2 > Threshold  SaturateOnIntegerOverflow=off  InputSameDT=off
  "T " : Outport
  wires:
  Failed?/1 -> Logical Operator/1
  Constant/1 -> Switch/1
  T/1 -> IsNaN/1, IsInf/1, Switch/3
  Switch/1 -> "T "/1
  Logical Operator/1 -> Switch/2
  IsNaN/1 -> Logical Operator/2
  IsInf/1 -> Logical Operator/3

== system Lib_EMTAT/Components/Power Flow/Resistive Load Bank/Failure Determination ==
  Fail? : Inport
  OCFail : Outport
  wires:
  Fail?/1 -> OCFail/1

== system Lib_EMTAT/Components/Power Flow/Resistive Load Bank/Fix Divide By Zero. ==
  I^2 : Inport
  abs(Pset) : Inport  Port=2
  Constant : Constant  Value=eps
  Divide1 : Product  Inputs=/*
  If the square of the current is not equal to zero. : Switch  Criteria=u2 ~= 0  SaturateOnIntegerOverflow=off  InputSameDT=off
  R : Outport
  wires:
  Divide1/1 -> R/1
  abs(Pset)/1 -> Divide1/2
  I^2/1 -> If the square of the current is not equal to zero./2, If the square of the current is not equal to zero./1
  Constant/1 -> If the square of the current is not equal to zero./3
  If the square of the current is not equal to zero./1 -> Divide1/1

== system Lib_EMTAT/Components/Power Flow/Resistive Load Bank/Fix Divide By Zero.1 ==
  V : Inport
  Pset : Inport  Port=2
  Constant : Constant  Value=eps
  Divide1 : Product  Inputs=/*
  If voltage is not equal to zero. : Switch  Criteria=u2 ~= 0  SaturateOnIntegerOverflow=off  InputSameDT=off
  I : Outport
  wires:
  V/1 -> If voltage is not equal to zero./1, If voltage is not equal to zero./2
  Pset/1 -> Divide1/2
  Divide1/1 -> I/1
  Constant/1 -> If voltage is not equal to zero./3
  If voltage is not equal to zero./1 -> Divide1/1

== system Lib_EMTAT/Components/Power Flow/Resistive Load Bank/Open Circuit Failure - Line to Neutral Voltage ==
  Failed? : Inport
  I : Inport  Port=2
  Constant : Constant  Value=0
  IsInf : RelationalOperator  Operator=isInf  OutDataTypeStr=boolean  RndMeth=Simplest  InputSameDT=off
  IsNaN : RelationalOperator  Operator=isNaN  OutDataTypeStr=boolean  RndMeth=Simplest  InputSameDT=off
  Logical Operator : Logic  Operator=OR  Inputs=3  AllPortsSameDT=off  OutDataTypeStr=boolean
  Switch : Switch  Criteria=u2 > Threshold  SaturateOnIntegerOverflow=off  InputSameDT=off
  "I " : Outport
  wires:
  Failed?/1 -> Logical Operator/1
  Constant/1 -> Switch/1
  I/1 -> IsNaN/1, IsInf/1, Switch/3
  Switch/1 -> "I "/1
  Logical Operator/1 -> Switch/2
  IsNaN/1 -> Logical Operator/2
  IsInf/1 -> Logical Operator/3

== system Lib_EMTAT/Components/Power Flow/Supercapacitor/SOC ==
  Energy (W-h) : Inport
  Divide : Product  Inputs=*/
  Gain : Gain  Gain=100
  Total Stored Energy (W-h) : Constant  Value=TSE
  SOC : Outport
  wires:
  Gain/1 -> SOC/1
  Divide/1 -> Gain/1
  Total Stored Energy (W-h)/1 -> Divide/2
  Energy (W-h)/1 -> Divide/1

== system Lib_EMTAT/Components/Power Flow/Supercapacitor/Voltage, V to Energy, Wh ==
  V : Inport
  Gain2 : Gain  Gain=0.5*C
  J to Wh : Gain  Gain=0.000277778
  Square : Math  Operator=square
  E : Outport
  wires:
  V/1 -> Square/1
  Gain2/1 -> J to Wh/1
  Square/1 -> Gain2/1
  J to Wh/1 -> E/1
